simulink model "Current_test"  (R2022a)
settings: Solver=ode1  StartTime=0.0  StopTime=inf  FixedStep=0.001  RelTol=1e-3  EnableMultiTasking=on
undefined symbols (not defined in the file): a, b, D, J, k1, k2, kd2, kd4, kii, kp2, kp4, kpi, kpo, Kt, L, R, Tc
libraries: arduinolib x21, arduinosensorlib x6, simulink_extras x2
settings Model: SimulationMode=external  ExtModeTrigDuration=2  Creator=LabPC  LastModifiedBy=LabPC
settings OptimizationCC: EnhancedBackFolding=on  PassReuseOutputArgsAs=Individual arguments  ZeroExternalMemoryAtStartup=off  ZeroInternalMemoryAtStartup=off  MaxStackSize=64  OptimizeBlockOrder=speed  DifferentSizesBufferReuse=on  OptimizationCustomize=off  EfficientTunableParamExpr=on
settings DebuggingCC: MultiTaskRateTransMsg=warning  ParameterTunabilityLossMsg=error
settings HardwareCC: ProdBitPerInt=16  ProdBitPerPointer=16  ProdBitPerSizeT=16  ProdBitPerPtrDiffT=16  ProdLargestAtomicFloat=None  ProdWordSize=8  ProdHWDeviceType=Atmel->AVR
settings SFSimCC: MATLABDynamicMemAlloc=off
settings RTWCC: SystemTargetFile=ert.tlc  HardwareBoard=Arduino Mega 2560  TemplateMakefile=ert_default_tmf  Toolchain=Arduino AVR  BuildConfiguration=Faster Runs
settings CodeAppCC: ForceParamTrailComments=on  IgnoreCustomStorageClasses=off  OperatorAnnotations=on  SimulinkDataObjDesc=on  SFDataObjDesc=on  InsertBlockDesc=on
settings ERTTargetCC: SupportContinuousTime=on  SupportVariableSizeSignals=on  ExtMode=on  ExtModeTransport=3  ExtModeStaticAlloc=on  ExtModeStaticAllocSize=2048  ExtModeMexFile=ext_xcp  ExtModeMexArgs=0 3 115200  ExtModeIntrfLevel=Level2 - Open

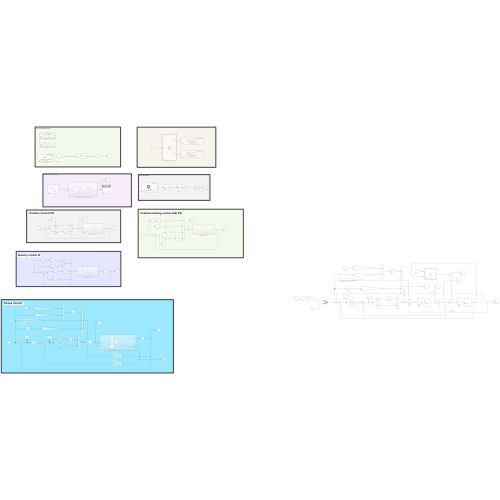
[thumbnail: Simulink's stored preview of the top-level diagram]
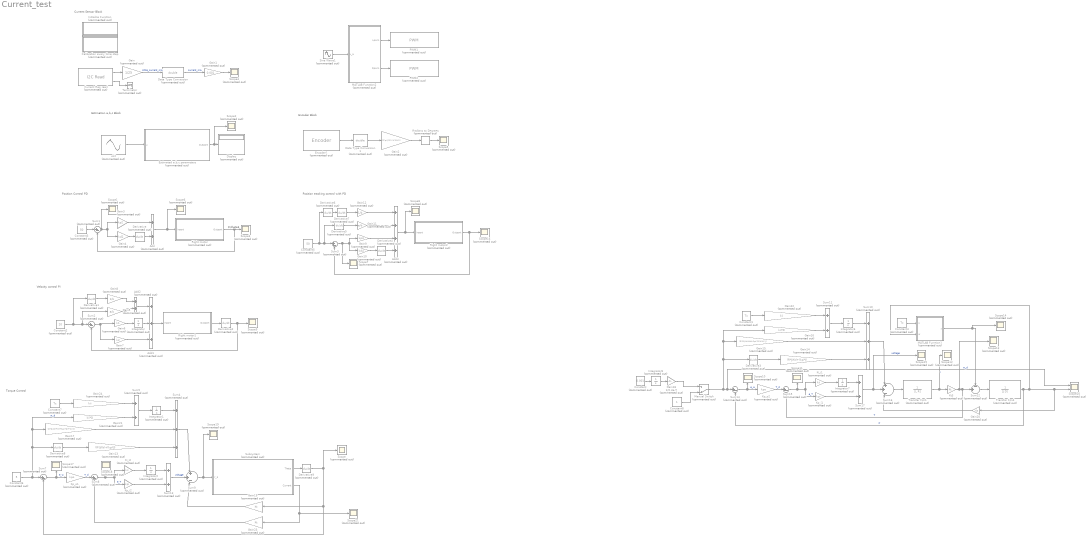
== system Current_test ==
  note: Current Sensor Block
  note: Encoder Block
  note: Estimation a,b,c Block
  note: $\theta$
  note: Position tracking control with PD
  note: Velocity control PI
  note: Torque Control
  note: Position Control PD
  Add : Sum  Commented=on
  Add1 : Sum  Commented=on  Inputs=+++
  Add2 : Sum  Commented=on
  Add3 : Sum  Commented=on  Inputs=++++
  Calibration every time step : Subsystem  Priority=0  Commented=on
  Constant : Constant  Commented=on  Value=0.001
  Constant1 : Constant  Commented=on  Value=Tc
  Constant2 : Constant  Commented=on  Value=20
  Constant3 : Constant  Commented=on  Value=50
  Constant4 : Constant  Commented=on  Value=Tc
  Constant5 : Constant  Commented=on  Value=50
  Constant6 : Constant  Commented=on  Value=5
  Constant7 : Constant  Commented=on  Value=Tc
  Constant8 : Constant  Commented=on
  Current Reg read : arduinolib/I2C Read  Commented=on  I2CModule=0  Mode=Master  SlaveAddress="hex2dec(\"0x40\")"  SlaveByteOrder=BigEndian  Direction=Receiver  RegisterAddressMode=on  RegisterAddress="hex2dec(\"0x04\")"  SlaveDataType=int16  DataLength=1  NoAck=off  RepeatedStart=off  OutputStatus=on  blockPlatform=ARDUINO  SampleTime=0.1
      settings: SourceProductBaseCode=ARDUINO
  Data Type Conversion : DataTypeConversion  Commented=on  OutDataTypeStr=double  SaturateOnIntegerOverflow=off  RndMeth=Floor
  Data Type Conversion1 : DataTypeConversion  Commented=on  OutDataTypeStr=double  SaturateOnIntegerOverflow=off  RndMeth=Floor
  Derivative{,1..9} (10 alike) : Derivative  Commented=on
  Display : Display  Commented=on
  Encoder1 : arduinosensorlib/Encoder  Commented=on  InputA=2  InputB=3  Mode=No reset  SampleTime=-1
      settings: SourceProductBaseCode=ARDUINO
  Estimated a,b,c parameters : Subsystem  Commented=on
  Gain : Gain  Commented=on  Gain=1/25
  Gain1 : Gain  Commented=on  Gain=0.001
  Gain10 : Gain  Commented=on  Gain=kd4
  Gain11 : Gain  Commented=on  Gain=a/b
  Gain12 : Gain  Commented=on  Gain=1/b
  Gain13 : Gain  Commented=on  Gain=(R*J/Kt)+(kpi*J)
  Gain14 : Gain  Commented=on  Gain=(R*J/Kt)+(kpi*J)
  Gain15 : Gain  Commented=on  Gain=(R*D/Kt)+Kt+(kpi*D)+(kii*J)
  Gain16 : Gain  Commented=on  Gain=kii*D
  Gain17 : Gain  Commented=on  Gain=(R*D/Kt)+Kt+(kpi*D)+(kii*J)
  Gain18 : Gain  Commented=on  Gain=1/0.3e-5
  Gain19 : Gain  Commented=on  Gain=Kt
  Gain2 : Gain  Commented=on  Gain=(2*pi)/(11*4*19.2)
  Gain20 : Gain  Commented=on  Gain=Kt
  Gain21 : Gain  Commented=on  Gain=kii*D
  Gain22 : Gain  Commented=on  Gain=kii
  Gain23 : Gain  Commented=on  Gain=Kt
  Gain24 : Gain  Commented=on  Gain=kii
  Gain3 : Gain  Commented=on  Gain=kp2
  Gain4 : Gain  Commented=on  Gain=kd2
  Gain5 : Gain  Commented=on  Gain=a/b
  Gain6 : Gain  Commented=on  Gain=k1
  Gain7 : Gain  Commented=on  Gain=k2
  Gain8 : Gain  Commented=on  Gain=1/b
  Gain9 : Gain  Commented=on  Gain=kp4
  Initialize Function : Subsystem  Commented=on  TreatAsAtomicUnit=on
  Integrator{,1..2,6..8} (6 alike) : Integrator  Commented=on
  Ki_i1 : Gain  Commented=on  Gain=kii
  Ki_i2 : Gain  Commented=on  Gain=kii
  Kp_i1 : Gain  Commented=on  Gain=kpi
  Kp_i2 : Gain  Commented=on  Gain=kpi
  Kp_o1 : Gain  Commented=on  Gain=kpo
  Kp_o2 : Gain  Commented=on  Gain=kpo
  Kt3 : Gain  Commented=on  Gain=Kt
  MATLAB Function1 : MATLAB Function  Commented=on  TreatAsAtomicUnit=on
  MATLAB Function2 : MATLAB Function  Commented=on  TreatAsAtomicUnit=on
  Manual Switch : ManualSwitch  Commented=on  CurrentSetting=0
  PWM1 : arduinolib/PWM  Commented=on  pinNumber=8  frequencyType=Default  desiredFrequency=490.2  achievableFrequency=490.2
  PWM2 : arduinolib/PWM  Commented=on  pinNumber=9  frequencyType=Default  desiredFrequency=490.2  achievableFrequency=490.2
  Radians to Degrees : simulink_extras/Transformations/Radians to Degrees  Commented=on
  Right motor : Subsystem  Commented=on
  Right motor1 : Subsystem  Commented=on
  Right motor2 : Subsystem  Commented=on
  Scope{,1..19,21} (21 alike) : Scope  Commented=on
  Scope20 : Scope  Commented=on  NumInputPorts=2
  Sine Wave1 : Sin  Commented=on  Amplitude=16  Frequency=0.5  SampleTime=0
  Subsystem : Subsystem  Commented=on
  Sum{1..3,7..8,14..15} (7 alike) : Sum  Commented=on  Inputs=|+-
  Sum10 : Sum  Commented=on  Inputs=+++
  Sum{5,11,13,17} (4 alike) : Sum  Commented=on
  Sum12 : Sum  Commented=on  Inputs=-|+||
  Sum16 : Sum  Commented=on  Inputs=|+|+|-|
  Sum4 : Sum  Commented=on  Inputs=+++
  Sum9 : Sum  Commented=on  Inputs=|+|+|-|
  Terminator : Terminator  Commented=on
  Transfer Fcn1 : TransferFcn  Commented=on  Denominator=[L R]
  Transfer Fcn4 : TransferFcn  Commented=on  Denominator=[J D]
  uk2 : Sin  Commented=on  Amplitude=14  Frequency=2*pi*1  SampleTime=0
  wires:
  MATLAB Function2/2(Rpwm) -> PWM2/1
  MATLAB Function2/1(Lpwm) -> PWM1/1
  Current Reg read/2 -> Terminator/1
  Gain/1 -> Data Type Conversion/1  "int16_current_mA"
  Current Reg read/1 -> Gain/1
  Sine Wave1/1 -> MATLAB Function2/1(v_a)
  Data Type Conversion/1 -> Gain1/1  "current_mA"
  Gain1/1 -> Scope4/1
  Gain2/1 -> Radians to Degrees/1
  Data Type Conversion1/1 -> Gain2/1
  Encoder1/1 -> Data Type Conversion1/1
  Radians to Degrees/1 -> Scope5/1
  Estimated a,b,c parameters/1(Outport) -> Scope2/1, Display/1
  uk2/1 -> Estimated a,b,c parameters/1(u)
  Constant3/1 -> Sum1/1
  Derivative/1 -> Add/2
  Gain3/1 -> Add/1
  Gain4/1 -> Derivative/1
  Right motor/1(Outport) -> Sum1/2, Scope3/1
  Sum1/1 -> Scope1/1, Gain4/1, Gain3/1
  Add/1 -> Right motor/1(Inport), Scope6/1
  Gain12/1 -> Add3/1
  Derivative5/1 -> Gain11/1
  Right motor2/1(Outport) -> Sum3/2, Scope16/1
  Add3/1 -> Scope8/1, Right motor2/1(Inport)
  Gain10/1 -> Derivative4/1
  Derivative7/1 -> Gain12/1
  Gain9/1 -> Add3/3
  Gain11/1 -> Add3/2
  Constant5/1 -> Derivative6/1, Derivative5/1, Sum3/1
  Derivative4/1 -> Add3/4
  Sum3/1 -> Scope7/1, Gain9/1, Gain10/1
  Derivative6/1 -> Derivative7/1
  Gain5/1 -> Add2/2
  Right motor1/1(Outport) -> Derivative2/1
  Derivative2/1 -> Scope9/1, Sum2/2
  Constant2/1 -> Gain5/1, Sum2/1, Derivative1/1
  Integrator/1 -> Add1/2
  Gain8/1 -> Add2/1
  Gain7/1 -> Add1/3
  Add2/1 -> Add1/1
  Gain6/1 -> Integrator/1
  Sum2/1 -> Gain6/1, Gain7/1
  Add1/1 -> Right motor1/1(Inport)
  Derivative1/1 -> Gain8/1
  Ki_i2/1 -> Integrator2/1
  Sum4/1 -> Sum9/1
  Sum5/1 -> Integrator1/1
  Derivative8/1 -> Gain13/1
  Gain17/1 -> Sum4/2
  Sum8/1 -> Scope18/1, Kp_i2/1, Ki_i2/1  "e_T"
  Kp_i2/1 -> Sum13/2
  Constant7/1 -> Gain24/1
  Integrator1/1 -> Sum4/1
  Gain24/1 -> Sum5/1
  Kp_o1/1 -> Sum8/1  "T_d"
  Sum13/1 -> Sum9/2  "voltage"
  Gain21/1 -> Sum5/2
  Sum7/1 -> Kp_o1/1, Scope17/1  "e_w"
  Integrator2/1 -> Sum13/1
  Constant6/1 -> Sum7/1, Derivative8/1, Gain17/1, Gain21/1  "w_d"
  Gain13/1 -> Sum4/3
  MATLAB Function1/1(y) -> Sum12/1, Scope14/1
  Sum14/1 -> Scope10/1, Kp_o2/1  "e_w"
  Constant4/1 -> MATLAB Function1/1(u)
  Sum16/1 -> Transfer Fcn1/1
  Sum12/1 -> Transfer Fcn4/1
  Integrator6/1 -> Sum10/1
  Sum15/1 -> Ki_i1/1, Kp_i1/1, Scope11/1  "e_T"
  Transfer Fcn1/1 -> Scope12/1, Kt3/1  "i"
  Manual Switch/1 -> Gain16/1, Gain15/1, Derivative3/1, Scope20/1, Sum14/1  "w_d"
  Gain20/1 -> Sum16/3
  Transfer Fcn4/1 -> Sum14/2, MATLAB Function1/2(w), Scope20/2, Gain20/1  "w"
  Integrator7/1 -> Sum17/1
  Sum10/1 -> Sum16/1
  Kt3/1 -> Scope13/1, Sum15/2, Sum12/2  "T"
  Gain14/1 -> Sum10/3
  Kp_o2/1 -> Sum15/1  "T_d"
  Integrator8/1 -> Gain18/1
  Sum11/1 -> Integrator6/1
  Gain22/1 -> Sum11/1
  Ki_i1/1 -> Integrator7/1
  Gain15/1 -> Sum10/2
  Derivative3/1 -> Gain14/1
  Constant1/1 -> Gain22/1
  Gain16/1 -> Sum11/2
  Sum17/1 -> Scope15/1, Sum16/2  "voltage"
  Kp_i1/1 -> Sum17/2
  Constant/1 -> Integrator8/1
  Constant8/1 -> Manual Switch/2
  Gain18/1 -> Manual Switch/1
  Sum9/1 -> Scope19/1, Subsystem/1(v_a)
  Subsystem/1(Theta) -> Derivative9/1
  Derivative9/1 -> Scope/1, Sum7/2, Gain19/1
  Gain19/1 -> Sum9/3
  Subsystem/2(Current) -> Gain23/1, Scope21/1
  Gain23/1 -> Sum8/2

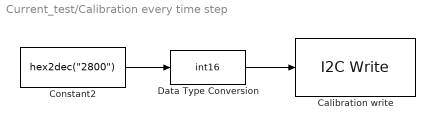
== system Current_test/Calibration every time step ==
  Calibration write : arduinolib/I2C Write  I2CModule=0  Mode=Master  SlaveAddress="uint8(hex2dec(\"0x40\"))"  SlaveByteOrder=BigEndian  Direction=Transmitter  RegisterAddressMode=on  RegisterAddress="uint8(hex2dec(\"0x05\"))"  SlaveDataType=uint8  DataLength=1  NoAck=off  RepeatedStart=off  OutputStatus=off  blockPlatform=ARDUINO
      settings: SourceProductBaseCode=ARDUINO
  Constant2 : Constant  Value="hex2dec(\"2800\")"
  Data Type Conversion : DataTypeConversion  OutDataTypeStr=int16  SaturateOnIntegerOverflow=off  RndMeth=Floor
  wires:
  Constant2/1 -> Data Type Conversion/1
  Data Type Conversion/1 -> Calibration write/1

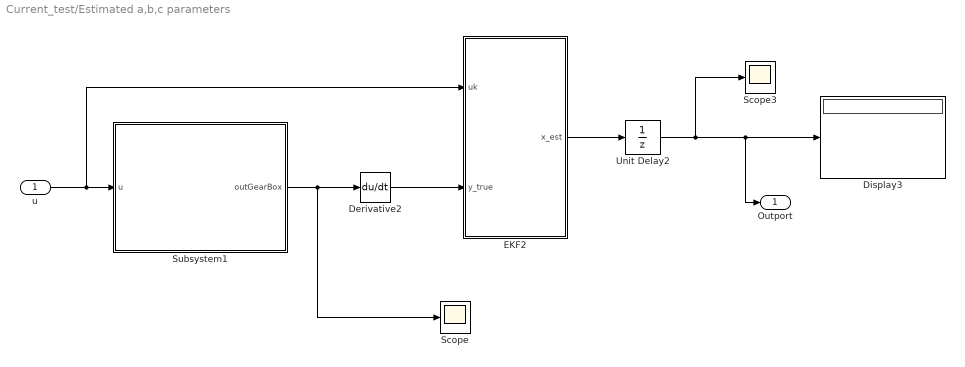
== system Current_test/Estimated a,b,c parameters ==
  u : Inport
  Derivative2 : Derivative
  Display3 : Display
  EKF2 : MATLAB Function  TreatAsAtomicUnit=on
  Scope : Scope
  Scope3 : Scope
  Subsystem1 : Subsystem
  Unit Delay2 : UnitDelay  InitialCondition=[0;0;0;0]  SampleTime=-1  HasFrameUpgradeWarning=on
  Outport : Outport
  wires:
  Derivative2/1 -> EKF2/2(y_true)
  Unit Delay2/1 -> Outport/1, Display3/1, Scope3/1
  EKF2/1(x_est) -> Unit Delay2/1
  Subsystem1/1(outGearBox) -> Scope/1, Derivative2/1
  u/1 -> EKF2/1(uk), Subsystem1/1(u)

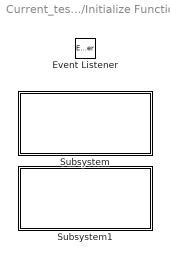
== system Current_test/Initialize Function ==
  Event Listener : EventListener  DisableCoverage=on  EventName=reset
  Subsystem : Subsystem  Priority=0
  Subsystem1 : Subsystem  Priority=1

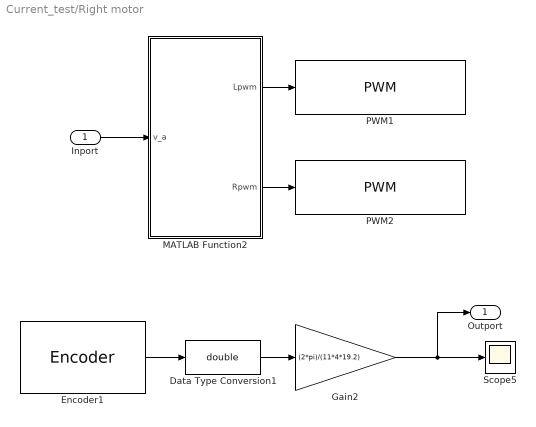
== system Current_test/Right motor ==
  Inport : Inport
  Data Type Conversion1 : DataTypeConversion  OutDataTypeStr=double  SaturateOnIntegerOverflow=off  RndMeth=Floor
  Encoder1 : arduinosensorlib/Encoder  InputA=2  InputB=3  Mode=No reset  SampleTime=-1
      settings: SourceProductBaseCode=ARDUINO
  Gain2 : Gain  Gain=(2*pi)/(11*4*19.2)
  MATLAB Function2 : MATLAB Function  TreatAsAtomicUnit=on
  PWM1 : arduinolib/PWM  pinNumber=8  frequencyType=Default  desiredFrequency=490.2  achievableFrequency=490.2
  PWM2 : arduinolib/PWM  pinNumber=9  frequencyType=Default  desiredFrequency=490.2  achievableFrequency=490.2
  Scope5 : Scope
  Outport : Outport
  wires:
  MATLAB Function2/2(Rpwm) -> PWM2/1
  MATLAB Function2/1(Lpwm) -> PWM1/1
  Inport/1 -> MATLAB Function2/1(v_a)
  Encoder1/1 -> Data Type Conversion1/1
  Data Type Conversion1/1 -> Gain2/1
  Gain2/1 -> Outport/1, Scope5/1

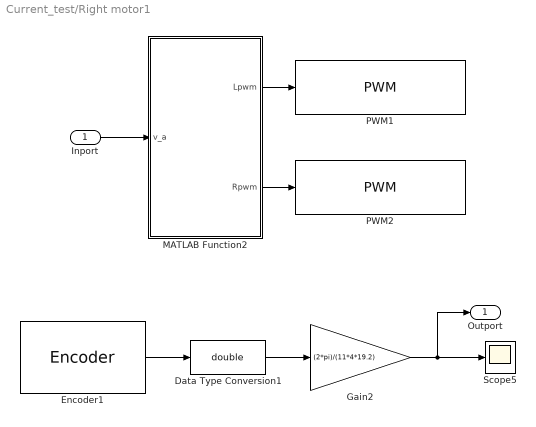
== system Current_test/Right motor1 ==
  Inport : Inport
  Data Type Conversion1 : DataTypeConversion  OutDataTypeStr=double  SaturateOnIntegerOverflow=off  RndMeth=Floor
  Encoder1 : arduinosensorlib/Encoder  InputA=2  InputB=3  Mode=No reset  SampleTime=-1
      settings: SourceProductBaseCode=ARDUINO
  Gain2 : Gain  Gain=(2*pi)/(11*4*19.2)
  MATLAB Function2 : MATLAB Function  TreatAsAtomicUnit=on
  PWM1 : arduinolib/PWM  pinNumber=8  frequencyType=Default  desiredFrequency=490.2  achievableFrequency=490.2
  PWM2 : arduinolib/PWM  pinNumber=9  frequencyType=Default  desiredFrequency=490.2  achievableFrequency=490.2
  Scope5 : Scope
  Outport : Outport
  wires:
  Gain2/1 -> Scope5/1, Outport/1
  Data Type Conversion1/1 -> Gain2/1
  Encoder1/1 -> Data Type Conversion1/1
  Inport/1 -> MATLAB Function2/1(v_a)
  MATLAB Function2/1(Lpwm) -> PWM1/1
  MATLAB Function2/2(Rpwm) -> PWM2/1

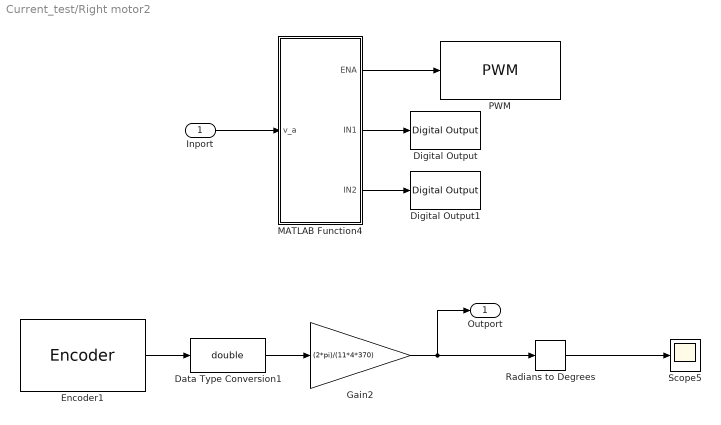
== system Current_test/Right motor2 ==
  Inport : Inport
  Data Type Conversion1 : DataTypeConversion  OutDataTypeStr=double  SaturateOnIntegerOverflow=off  RndMeth=Floor
  Digital Output : arduinolib/Digital Output  pinNumber=5  Direction=output  blockPlatform=arduino
  Digital Output1 : arduinolib/Digital Output  pinNumber=7  Direction=output  blockPlatform=arduino
  Encoder1 : arduinosensorlib/Encoder  InputA=2  InputB=3  Mode=No reset  SampleTime=-1
      settings: SourceProductBaseCode=ARDUINO
  Gain2 : Gain  Gain=(2*pi)/(11*4*370)
  MATLAB Function4 : MATLAB Function  TreatAsAtomicUnit=on
  PWM : arduinolib/PWM  pinNumber=4  frequencyType=Default  desiredFrequency=490.2  achievableFrequency=490.2
  Radians to Degrees : simulink_extras/Transformations/Radians to Degrees
  Scope5 : Scope
  Outport : Outport
  wires:
  Gain2/1 -> Radians to Degrees/1, Outport/1
  Data Type Conversion1/1 -> Gain2/1
  Encoder1/1 -> Data Type Conversion1/1
  MATLAB Function4/1(ENA) -> PWM/1
  MATLAB Function4/2(IN1) -> Digital Output/1
  MATLAB Function4/3(IN2) -> Digital Output1/1
  Inport/1 -> MATLAB Function4/1(v_a)
  Radians to Degrees/1 -> Scope5/1

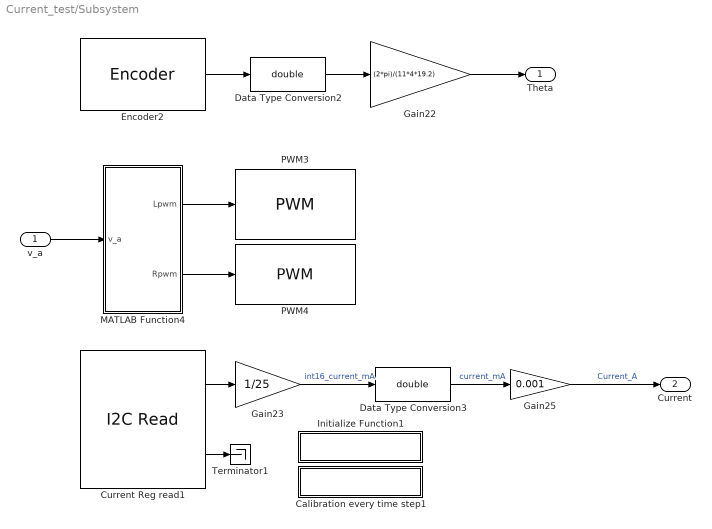
== system Current_test/Subsystem ==
  v_a : Inport
  Calibration every time step1 : Subsystem  Priority=0
  Current Reg read1 : arduinolib/I2C Read  I2CModule=0  Mode=Master  SlaveAddress="hex2dec(\"0x40\")"  SlaveByteOrder=BigEndian  Direction=Receiver  RegisterAddressMode=on  RegisterAddress="hex2dec(\"0x04\")"  SlaveDataType=int16  DataLength=1  NoAck=off  RepeatedStart=off  OutputStatus=on  blockPlatform=ARDUINO  SampleTime=0.1
      settings: SourceProductBaseCode=ARDUINO
  Data Type Conversion2 : DataTypeConversion  OutDataTypeStr=double  SaturateOnIntegerOverflow=off  RndMeth=Floor
  Data Type Conversion3 : DataTypeConversion  OutDataTypeStr=double  SaturateOnIntegerOverflow=off  RndMeth=Floor
  Encoder2 : arduinosensorlib/Encoder  InputA=2  InputB=3  Mode=No reset  SampleTime=-1
      settings: SourceProductBaseCode=ARDUINO
  Gain22 : Gain  Gain=(2*pi)/(11*4*19.2)
  Gain23 : Gain  Gain=1/25
  Gain25 : Gain  Gain=0.001
  Initialize Function1 : Subsystem  TreatAsAtomicUnit=on
  MATLAB Function4 : MATLAB Function  TreatAsAtomicUnit=on
  PWM3 : arduinolib/PWM  pinNumber=8  frequencyType=Default  desiredFrequency=490.2  achievableFrequency=490.2
  PWM4 : arduinolib/PWM  pinNumber=9  frequencyType=Default  desiredFrequency=490.2  achievableFrequency=490.2
  Terminator1 : Terminator
  Theta : Outport
  Current : Outport  Port=2
  wires:
  Current Reg read1/2 -> Terminator1/1
  Data Type Conversion3/1 -> Gain25/1  "current_mA"
  Gain23/1 -> Data Type Conversion3/1  "int16_current_mA"
  Data Type Conversion2/1 -> Gain22/1
  Encoder2/1 -> Data Type Conversion2/1
  MATLAB Function4/1(Lpwm) -> PWM3/1
  MATLAB Function4/2(Rpwm) -> PWM4/1
  Current Reg read1/1 -> Gain23/1
  Gain22/1 -> Theta/1
  v_a/1 -> MATLAB Function4/1(v_a)
  Gain25/1 -> Current/1  "Current_A"

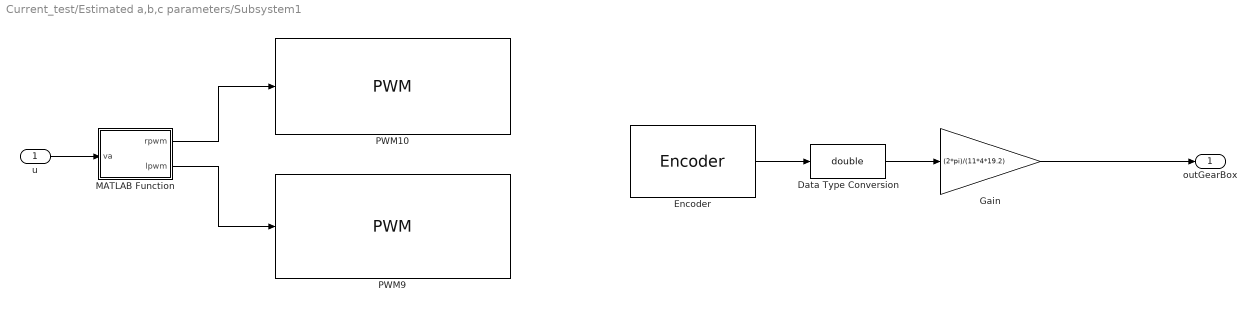
== system Current_test/Estimated a,b,c parameters/Subsystem1 ==
  u : Inport
  Data Type Conversion : DataTypeConversion  OutDataTypeStr=double  SaturateOnIntegerOverflow=off  RndMeth=Floor
  Encoder : arduinosensorlib/Encoder  InputA=2  InputB=3  Mode=No reset  SampleTime=-1
      settings: SourceProductBaseCode=ARDUINO
  Gain : Gain  Gain=(2*pi)/(11*4*19.2)
  MATLAB Function : MATLAB Function  TreatAsAtomicUnit=on
  PWM10 : arduinolib/PWM  pinNumber=8  frequencyType=Default  desiredFrequency=490.2  achievableFrequency=490.2
  PWM9 : arduinolib/PWM  pinNumber=9  frequencyType=Default  desiredFrequency=490.2  achievableFrequency=490.2
  outGearBox : Outport
  wires:
  Gain/1 -> outGearBox/1
  u/1 -> MATLAB Function/1(va)
  MATLAB Function/1(rpwm) -> PWM10/1
  MATLAB Function/2(lpwm) -> PWM9/1
  Encoder/1 -> Data Type Conversion/1
  Data Type Conversion/1 -> Gain/1

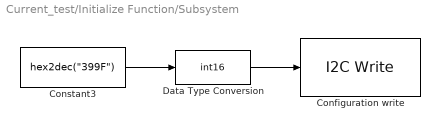
== system Current_test/Initialize Function/Subsystem ==
  Configuration write : arduinolib/I2C Write  I2CModule=0  Mode=Master  SlaveAddress="hex2dec(\"0x40\")"  SlaveByteOrder=BigEndian  Direction=Transmitter  RegisterAddressMode=on  RegisterAddress="hex2dec(\"0x00\")"  SlaveDataType=uint8  DataLength=1  NoAck=off  RepeatedStart=off  OutputStatus=off  blockPlatform=ARDUINO
      settings: SourceProductBaseCode=ARDUINO
  Constant3 : Constant  Value="hex2dec(\"399F\")"
  Data Type Conversion : DataTypeConversion  OutDataTypeStr=int16  SaturateOnIntegerOverflow=off  RndMeth=Floor
  wires:
  Constant3/1 -> Data Type Conversion/1
  Data Type Conversion/1 -> Configuration write/1

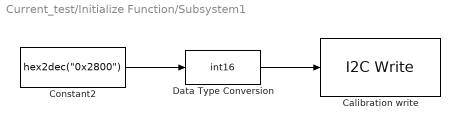
== system Current_test/Initialize Function/Subsystem1 ==
  Calibration write : arduinolib/I2C Write  I2CModule=0  Mode=Master  SlaveAddress="uint8(hex2dec(\"0x40\"))"  SlaveByteOrder=BigEndian  Direction=Transmitter  RegisterAddressMode=on  RegisterAddress="uint8(hex2dec(\"0x05\"))"  SlaveDataType=uint8  DataLength=1  NoAck=off  RepeatedStart=off  OutputStatus=off  blockPlatform=ARDUINO
      settings: SourceProductBaseCode=ARDUINO
  Constant2 : Constant  Value="hex2dec(\"0x2800\")"
  Data Type Conversion : DataTypeConversion  OutDataTypeStr=int16  SaturateOnIntegerOverflow=off  RndMeth=Floor
  wires:
  Constant2/1 -> Data Type Conversion/1
  Data Type Conversion/1 -> Calibration write/1

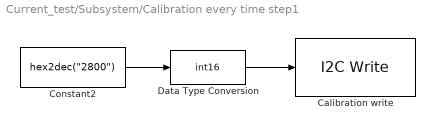
== system Current_test/Subsystem/Calibration every time step1 ==
  Calibration write : arduinolib/I2C Write  I2CModule=0  Mode=Master  SlaveAddress="uint8(hex2dec(\"0x40\"))"  SlaveByteOrder=BigEndian  Direction=Transmitter  RegisterAddressMode=on  RegisterAddress="uint8(hex2dec(\"0x05\"))"  SlaveDataType=uint8  DataLength=1  NoAck=off  RepeatedStart=off  OutputStatus=off  blockPlatform=ARDUINO
      settings: SourceProductBaseCode=ARDUINO
  Constant2 : Constant  Value="hex2dec(\"2800\")"
  Data Type Conversion : DataTypeConversion  OutDataTypeStr=int16  SaturateOnIntegerOverflow=off  RndMeth=Floor
  wires:
  Data Type Conversion/1 -> Calibration write/1
  Constant2/1 -> Data Type Conversion/1

== system Current_test/Subsystem/Initialize Function1 ==
  Event Listener : EventListener  DisableCoverage=on  EventName=reset
  Subsystem : Subsystem  Priority=0
  Subsystem1 : Subsystem  Priority=1

== system Current_test/Subsystem/Initialize Function1/Subsystem ==
  Configuration write : arduinolib/I2C Write  I2CModule=0  Mode=Master  SlaveAddress="hex2dec(\"0x40\")"  SlaveByteOrder=BigEndian  Direction=Transmitter  RegisterAddressMode=on  RegisterAddress="hex2dec(\"0x00\")"  SlaveDataType=uint8  DataLength=1  NoAck=off  RepeatedStart=off  OutputStatus=off  blockPlatform=ARDUINO
      settings: SourceProductBaseCode=ARDUINO
  Constant3 : Constant  Value="hex2dec(\"399F\")"
  Data Type Conversion : DataTypeConversion  OutDataTypeStr=int16  SaturateOnIntegerOverflow=off  RndMeth=Floor
  wires:
  Data Type Conversion/1 -> Configuration write/1
  Constant3/1 -> Data Type Conversion/1

== system Current_test/Subsystem/Initialize Function1/Subsystem1 ==
  Calibration write : arduinolib/I2C Write  I2CModule=0  Mode=Master  SlaveAddress="uint8(hex2dec(\"0x40\"))"  SlaveByteOrder=BigEndian  Direction=Transmitter  RegisterAddressMode=on  RegisterAddress="uint8(hex2dec(\"0x05\"))"  SlaveDataType=uint8  DataLength=1  NoAck=off  RepeatedStart=off  OutputStatus=off  blockPlatform=ARDUINO
      settings: SourceProductBaseCode=ARDUINO
  Constant2 : Constant  Value="hex2dec(\"0x2800\")"
  Data Type Conversion : DataTypeConversion  OutDataTypeStr=int16  SaturateOnIntegerOverflow=off  RndMeth=Floor
  wires:
  Data Type Conversion/1 -> Calibration write/1
  Constant2/1 -> Data Type Conversion/1

== matlab function Current_test/MATLAB Function2 ==
  data: v_a input; Lpwm output; Rpwm output
function [Lpwm,Rpwm] = fcn(v_a)

vmax = 22.9;
pwm_cal = v_a*254/vmax;

if pwm_cal > 0
    Lpwm = 0;
    Rpwm = pwm_cal;
elseif pwm_cal < 0
    Lpwm = abs(pwm_cal);
    Rpwm = 0;
else
    Lpwm = 0;
    Rpwm = 0;
end

== matlab function Current_test/Estimated a,b,c parameters/EKF2 ==
  settings: updateMethod=DISCRETE
  data: uk input; y_true input; x_est output
function x_est = fcn(uk,y_true)
Ts=0.01;
persistent x_est_p P Qd_est R_est Qc_est;
if isempty(x_est_p)
          
          x_est_p=[2;13;25;1];
          P=2*eye(4);
         Qc_est=1e-5*diag([10,25,25,1]);
          Qd_est=Qc_est*Ts;
          R_est=0.02;
end
c=[1 0 0 0];D=0;Ck=c;Dk=D;
%Comput Kalman Gain and update predicted value
Wk=P*Ck'/(Ck*P*Ck'+R_est);
y_est=Ck*x_est_p+Dk*uk;
x=x_est_p+Wk.*(y_true-y_est);
%Compute prediction at next time step
x_est=x+Ts*[-x(2)*x(1)+uk*x(3)-x(4)*sign(x(1));0;0;0];
%Update error covariance matrices
P=P-Wk*Ck*P;
%Define Ak
Ak=eye(4)+Ts*[-x(2) -x(1) uk -sign(x(1));0 0 0 0;0 0 0 0;0 0 0 0];
P=Ak*P*Ak'+Qd_est;
x_est_p=x_est;

== matlab function Current_test/Estimated a,b,c parameters/Subsystem1/MATLAB Function ==
  data: va input; rpwm output; lpwm output
function [rpwm,lpwm] = fcn(va)

pwm = (va/24)*254;

if pwm > 0
    rpwm = pwm;
    lpwm = 0;
elseif pwm<0
    rpwm = 0;
    lpwm = abs(pwm);
else
    rpwm = 0;
    lpwm = 0;
end

== matlab function Current_test/Right motor/MATLAB Function2 ==
  data: v_a input; Lpwm output; Rpwm output
function [Lpwm,Rpwm] = fcn(v_a)

vmax = 22.9;
pwm_cal = v_a*254/vmax;

if pwm_cal > 0
    Lpwm = 0;
    Rpwm = pwm_cal;
elseif pwm_cal < 0
    Lpwm = abs(pwm_cal);
    Rpwm = 0;
else
    Lpwm = 0;
    Rpwm = 0;
end

== matlab function Current_test/Right motor1/MATLAB Function2 ==
  data: v_a input; Lpwm output; Rpwm output
function [Lpwm,Rpwm] = fcn(v_a)

vmax = 22.9;
pwm_cal = v_a*254/vmax;

if pwm_cal > 0
    Lpwm = 0;
    Rpwm = pwm_cal;
elseif pwm_cal < 0
    Lpwm = abs(pwm_cal);
    Rpwm = 0;
else
    Lpwm = 0;
    Rpwm = 0;
end

== matlab function Current_test/Subsystem/MATLAB Function4 ==
  data: v_a input; Lpwm output; Rpwm output
function [Lpwm,Rpwm] = fcn(v_a)

vmax = 22.9;
pwm_cal = v_a*254/vmax;

if pwm_cal > 0
    Lpwm = 0;
    Rpwm = pwm_cal;
elseif pwm_cal < 0
    Lpwm = abs(pwm_cal);
    Rpwm = 0;
else
    Lpwm = 0;
    Rpwm = 0;
end

== matlab function Current_test/Right motor2/MATLAB Function4 ==
  data: v_a input; ENA output; IN1 output; IN2 output
function [ENA,IN1,IN2] = fcn(v_a)

vmax = 12;
pwm_cal = v_a*254/vmax;

if pwm_cal > 0
   
    ENA = pwm_cal;
    IN1 = 1;
    IN2 = 0;
elseif pwm_cal < 0
   
    ENA = abs(pwm_cal);
    IN1 = 0;
    IN2 = 1;
else
    ENA = 0;
    IN1 = 0;
    IN2 = 0;
   
end

== matlab function Current_test/MATLAB Function1 ==
  data: u input; y output; w input
function y = fcn(u,w)

y = u*sign(w);
